simulink model "object_frame_impedance"  (R2025a)
settings: Solver=FixedStepDiscrete  StartTime=0.0  StopTime=inf  FixedStep=0.0315/(4*12)  RelTol=1e-3  EnableMultiTasking=on
undefined symbols (not defined in the file or in its folder): f_step, force_step, K_Conn, K_D, K_Or, K_Ot, K_P, ksi, Kx, l_des, Mo, Newton, qd_initial_touch, R_O_Desired, Raphson, sigbuilder_block, t_f_start, torque_step, x_O_desired
libraries: dspmtrx3 x33, dspinverses x1
(part 6 of 6)

== matlab function object_frame_impedance/Control/IPC/J/J_Or1/Embedded MATLAB Function2 ==
  data: xi input double size=[4 3]; J_r3 output
%#eml
function J_r3 = partial_r3_to_x(xi)


x1 = xi(1,:)';
x2 = xi(2,:)';
x3 = xi(3,:)';
x4 = xi(4,:)';

r1=(( x1-x3 )/norm( x1-x3 ) + ...
    ( x2-x4 )/norm( x2-x4 ));


r1_unit=(r1/norm(r1));

r3 = skew( x1-x3 ) * ( x2-x4 );
r3_unit=r3/norm(r3);

r2_unit = skew(r3_unit)*r1_unit;

% RO=[r1_unit r2_unit r3_unit];


% partial_r3__term1 = (((norm(r3)^2)*eye(3)-(r3)*(r3)') / (norm((r3))^3));
partial_r3__term1 = (-skew(r3)^2)/(norm(r3)^3);

partial_r3__term2_x1x3 = skew(x2-x4)';
partial_r3__term2_x2x4 =  skew(x1-x3); 

partial_r3__term3_x1x2 =  eye(3);
partial_r3__term3_x3x4 = -eye(3);

J_r3_x1 = partial_r3__term1*partial_r3__term2_x1x3*partial_r3__term3_x1x2;

J_r3_x2 = partial_r3__term1*partial_r3__term2_x2x4*partial_r3__term3_x1x2;
       
J_r3_x3 = partial_r3__term1*partial_r3__term2_x1x3*partial_r3__term3_x3x4;
                    
J_r3_x4 = partial_r3__term1*partial_r3__term2_x2x4*partial_r3__term3_x3x4;


J_r3 = [J_r3_x1,J_r3_x2,J_r3_x3,J_r3_x4];

== matlab function object_frame_impedance/Control/IPC/J/J_Or1/Embedded MATLAB Function3 ==
  data: xi input double size=[4 3]; J_r1 output
%#eml
function J_r1 = partial_r1_to_x(xi)


x1 = xi(1,:)';
x2 = xi(2,:)';
x3 = xi(3,:)';
x4 = xi(4,:)';

r1=(( x1-x3 )/norm( x1-x3 ) + ( x2-x4 )/norm( x2-x4 ));

% r1=(( x1-x3 )/norm( x1-x3 ) + ( x2-x4 ))


r1_unit=(r1/norm(r1));

r3= skew( x1-x3 ) * ( x2-x4 );
r3_unit=r3/norm(r3);

r2_unit = skew(r3_unit)*r1_unit;

% RO=[r1_unit r2_unit r3_unit];


% partial_r1__term1 = (((norm(r1)^2)*eye(3)-(r1)*(r1)') / (norm((r1))^3));
partial_r1__term1 = (-skew(r1)^2)/(norm(r1)^3);

partial_r1__term2_x1x3 = (((norm((x1-x3))^2)*eye(3)-(x1-x3)*(x1-x3)') / (norm((x1-x3))^3));
partial_r1__term2_x2x4 = (((norm((x2-x4))^2)*eye(3)-(x2-x4)*(x2-x4)') / (norm((x2-x4))^3));


partial_r1__term3_x1x2 = eye(3);
partial_r1__term3_x3x4 = -eye(3);



J_r1_x1 = partial_r1__term1*partial_r1__term2_x1x3*partial_r1__term3_x1x2;

J_r2 = skew(r3_unit)*J_r1_x1';

J_r1_x2 = partial_r1__term1*partial_r1__term2_x2x4*partial_r1__term3_x1x2;
       
J_r1_x3 = partial_r1__term1*partial_r1__term2_x1x3*partial_r1__term3_x3x4;
       
J_r1_x4 = partial_r1__term1*partial_r1__term2_x2x4*partial_r1__term3_x3x4;


% J_r1_x1 = [partial_r1__term1.*partial_r1__term2_x1x3.*partial_r1__term3_x1x2(:,1), ...
%            partial_r1__term1.*partial_r1__term2_x1x3.*partial_r1__term3_x1x2(:,2), ...
%            partial_r1__term1.*partial_r1__term2_x1x3.*partial_r1__term3_x1x2(:,3)];
% 
% J_r1_x2 = [partial_r1__term1.*partial_r1__term2_x2x4.*partial_r1__term3_x1x2(:,1), ...
%            partial_r1__term1.*partial_r1__term2_x2x4.*partial_r1__term3_x1x2(:,2), ...
%            partial_r1__term1.*partial_r1__term2_x2x4.*partial_r1__term3_x1x2(:,3)];
%        
% J_r1_x3 = [partial_r1__term1.*partial_r1__term2_x1x3.*partial_r1__term3_x3x4(:,1), ...
%            partial_r1__term1.*partial_r1__term2_x1x3.*partial_r1__term3_x3x4(:,2), ...
%            partial_r1__term1.*partial_r1__term2_x1x3.*partial_r1__term3_x3x4(:,3)];
%        
% J_r1_x4 = [partial_r1__term1.*partial_r1__term2_x2x4.*partial_r1__term3_x3x4(:,1), ...
%            partial_r1__term1.*partial_r1__term2_x2x4.*partial_r1__term3_x3x4(:,2), ...
%            partial_r1__term1.*partial_r1__term2_x2x4.*partial_r1__term3_x3x4(:,3)];

J_r1 = [J_r1_x1,J_r1_x2,J_r1_x3,J_r1_x4];

== matlab function object_frame_impedance/Control/IPC/Object Level Damping(theta)/Embedded MATLAB Function ==
  data: q input; M output
%#eml
function M=Inertia_Dynamic_Terms(q)

M1=zeros(16);

L1 = 0.10;
L2 = 1.10;
L3 = 0.60;
L4 = 0.55;

capsule1Inertia = 0.1675;
capsule2Inertia = 0.0837;
capsule3Inertia = 0.0834;

caspule1mass = 2.00;
caspule2mass = 1.00;
caspule3mass = 1.00;

for i=1:4:16,
q1 = q(i);
q2 = q(i+1);
q3 = q(i+2);
q4 = q(i+3);
    
    
M1(i:i+3,i:i+3)=[capsule1Inertia .* cos(q2) .^ 2 + capsule2Inertia .* cos(q2 + q3) ...
   .^ 2 + capsule3Inertia .* cos(q2 + q3 + q4) .^ 2 + caspule1mass  ...
  .* ((1 / 4) .* L2 .^ 2 .* cos(q1) .^ 2 .* cos(q2) .^ 2 + (1 / 4)  ...
  .* L2 .^ 2 .* cos(q2) .^ 2 .* sin(q1) .^ 2) + caspule2mass .* ((( ...
  -1 / 2) .* L3 .* cos(q1) .* cos(q2 + q3) + cos(q1) .* (L2 .* cos( ...
  q2) + L3 .* cos(q2 + q3))) .^ 2 + ((1 / 2) .* L3 .* cos(q2 + q3)  ...
  .* sin(q1) + (-1) .* (L2 .* cos(q2) + L3 .* cos(q2 + q3)) .* sin( ...
  q1)) .^ 2) + caspule3mass .* (((-1 / 2) .* L4 .* cos(q1) .* cos( ...
  q2 + q3 + q4) + cos(q1) .* (L2 .* cos(q2) + L3 .* cos(q2 + q3) +  ...
  L4 .* cos(q2 + q3 + q4))) .^ 2 + ((1 / 2) .* L4 .* cos(q2 + q3 +  ...
  q4) .* sin(q1) + (-1) .* (L2 .* cos(q2) + L3 .* cos(q2 + q3) + L4  ...
  .* cos(q2 + q3 + q4)) .* sin(q1)) .^ 2) + capsule1Inertia .* sin( ...
  q2) .^ 2 + capsule2Inertia .* sin(q2 + q3) .^ 2 + capsule3Inertia  ...
  .* sin(q2 + q3 + q4) .^ 2,caspule2mass .* ((-1) .* ((-1 / 2) .*  ...
  L3 .* cos(q1) .* cos(q2 + q3) + cos(q1) .* (L2 .* cos(q2) + L3 .*  ...
  cos(q2 + q3))) .* sin(q1) .* (L2 .* sin(q2) + (1 / 2) .* L3 .*  ...
  sin(q2 + q3)) + (-1) .* cos(q1) .* ((1 / 2) .* L3 .* cos(q2 + q3)  ...
  .* sin(q1) + (-1) .* (L2 .* cos(q2) + L3 .* cos(q2 + q3)) .* sin( ...
  q1)) .* (L2 .* sin(q2) + (1 / 2) .* L3 .* sin(q2 + q3))) +  ...
  caspule3mass .* ((-1) .* ((-1 / 2) .* L4 .* cos(q1) .* cos(q2 +  ...
  q3 + q4) + cos(q1) .* (L2 .* cos(q2) + L3 .* cos(q2 + q3) + L4 .*  ...
  cos(q2 + q3 + q4))) .* sin(q1) .* (L2 .* sin(q2) + L3 .* sin(q2 +  ...
  q3) + (1 / 2) .* L4 .* sin(q2 + q3 + q4)) + (-1) .* cos(q1) .* (( ...
  1 / 2) .* L4 .* cos(q2 + q3 + q4) .* sin(q1) + (-1) .* (L2 .* cos( ...
  q2) + L3 .* cos(q2 + q3) + L4 .* cos(q2 + q3 + q4)) .* sin(q1)) .* ...
   (L2 .* sin(q2) + L3 .* sin(q2 + q3) + (1 / 2) .* L4 .* sin(q2 +  ...
  q3 + q4))),caspule2mass .* ((-1 / 2) .* L3 .* ((-1 / 2) .* L3 .*  ...
  cos(q1) .* cos(q2 + q3) + cos(q1) .* (L2 .* cos(q2) + L3 .* cos( ...
  q2 + q3))) .* sin(q1) .* sin(q2 + q3) + (-1 / 2) .* L3 .* cos(q1)  ...
  .* ((1 / 2) .* L3 .* cos(q2 + q3) .* sin(q1) + (-1) .* (L2 .* cos( ...
  q2) + L3 .* cos(q2 + q3)) .* sin(q1)) .* sin(q2 + q3)) +  ...
  caspule3mass .* ((-1) .* ((-1 / 2) .* L4 .* cos(q1) .* cos(q2 +  ...
  q3 + q4) + cos(q1) .* (L2 .* cos(q2) + L3 .* cos(q2 + q3) + L4 .*  ...
  cos(q2 + q3 + q4))) .* sin(q1) .* (L3 .* sin(q2 + q3) + (1 / 2) .* ...
   L4 .* sin(q2 + q3 + q4)) + (-1) .* cos(q1) .* ((1 / 2) .* L4 .*  ...
  cos(q2 + q3 + q4) .* sin(q1) + (-1) .* (L2 .* cos(q2) + L3 .* cos( ...
  q2 + q3) + L4 .* cos(q2 + q3 + q4)) .* sin(q1)) .* (L3 .* sin(q2 + ...
   q3) + (1 / 2) .* L4 .* sin(q2 + q3 + q4))),caspule3mass .* ((-1  ...
  / 2) .* L4 .* ((-1 / 2) .* L4 .* cos(q1) .* cos(q2 + q3 + q4) +  ...
  cos(q1) .* (L2 .* cos(q2) + L3 .* cos(q2 + q3) + L4 .* cos(q2 +  ...
  q3 + q4))) .* sin(q1) .* sin(q2 + q3 + q4) + (-1 / 2) .* L4 .*  ...
  cos(q1) .* ((1 / 2) .* L4 .* cos(q2 + q3 + q4) .* sin(q1) + (-1)  ...
  .* (L2 .* cos(q2) + L3 .* cos(q2 + q3) + L4 .* cos(q2 + q3 + q4))  ...
  .* sin(q1)) .* sin(q2 + q3 + q4));caspule2mass .* ((-1) .* ((-1 /  ...
  2) .* L3 .* cos(q1) .* cos(q2 + q3) + cos(q1) .* (L2 .* cos(q2) +  ...
  L3 .* cos(q2 + q3))) .* sin(q1) .* (L2 .* sin(q2) + (1 / 2) .* L3  ...
  .* sin(q2 + q3)) + (-1) .* cos(q1) .* ((1 / 2) .* L3 .* cos(q2 +  ...
  q3) .* sin(q1) + (-1) .* (L2 .* cos(q2) + L3 .* cos(q2 + q3)) .*  ...
  sin(q1)) .* (L2 .* sin(q2) + (1 / 2) .* L3 .* sin(q2 + q3))) +  ...
  caspule3mass .* ((-1) .* ((-1 / 2) .* L4 .* cos(q1) .* cos(q2 +  ...
  q3 + q4) + cos(q1) .* (L2 .* cos(q2) + L3 .* cos(q2 + q3) + L4 .*  ...
  cos(q2 + q3 + q4))) .* sin(q1) .* (L2 .* sin(q2) + L3 .* sin(q2 +  ...
  q3) + (1 / 2) .* L4 .* sin(q2 + q3 + q4)) + (-1) .* cos(q1) .* (( ...
  1 / 2) .* L4 .* cos(q2 + q3 + q4) .* sin(q1) + (-1) .* (L2 .* cos( ...
  q2) + L3 .* cos(q2 + q3) + L4 .* cos(q2 + q3 + q4)) .* sin(q1)) .* ...
   (L2 .* sin(q2) + L3 .* sin(q2 + q3) + (1 / 2) .* L4 .* sin(q2 +  ...
  q3 + q4))),capsule1Inertia .* cos(q1) .^ 2 .* (cos(q1) .^ 2 + sin( ...
  q1) .^ 2) + capsule2Inertia .* cos(q1) .^ 2 .* (cos(q1) .^ 2 +  ...
  sin(q1) .^ 2) + capsule3Inertia .* cos(q1) .^ 2 .* (cos(q1) .^ 2 + ...
   sin(q1) .^ 2) + capsule1Inertia .* sin(q1) .^ 2 .* (cos(q1) .^ 2  ...
  + sin(q1) .^ 2) + capsule2Inertia .* sin(q1) .^ 2 .* (cos(q1) .^  ...
  2 + sin(q1) .^ 2) + capsule3Inertia .* sin(q1) .^ 2 .* (cos(q1)  ...
  .^ 2 + sin(q1) .^ 2) + caspule1mass .* (((1 / 2) .* L2 .* cos(q1)  ...
  .^ 2 .* cos(q2) + (1 / 2) .* L2 .* cos(q2) .* sin(q1) .^ 2) .^ 2 + ...
   (1 / 4) .* L2 .^ 2 .* cos(q1) .^ 2 .* sin(q2) .^ 2 + (1 / 4) .*  ...
  L2 .^ 2 .* sin(q1) .^ 2 .* sin(q2) .^ 2) + caspule2mass .* ((cos( ...
  q1) .* ((-1 / 2) .* L3 .* cos(q1) .* cos(q2 + q3) + cos(q1) .* ( ...
  L2 .* cos(q2) + L3 .* cos(q2 + q3))) + sin(q1) .* ((-1 / 2) .* L3  ...
  .* cos(q2 + q3) .* sin(q1) + (L2 .* cos(q2) + L3 .* cos(q2 + q3))  ...
  .* sin(q1))) .^ 2 + cos(q1) .^ 2 .* (L2 .* sin(q2) + (1 / 2) .*  ...
  L3 .* sin(q2 + q3)) .^ 2 + sin(q1) .^ 2 .* (L2 .* sin(q2) + (1 /  ...
  2) .* L3 .* sin(q2 + q3)) .^ 2) + caspule3mass .* ((cos(q1) .* (( ...
  -1 / 2) .* L4 .* cos(q1) .* cos(q2 + q3 + q4) + cos(q1) .* (L2 .*  ...
  cos(q2) + L3 .* cos(q2 + q3) + L4 .* cos(q2 + q3 + q4))) + sin(q1) ...
   .* ((-1 / 2) .* L4 .* cos(q2 + q3 + q4) .* sin(q1) + (L2 .* cos( ...
  q2) + L3 .* cos(q2 + q3) + L4 .* cos(q2 + q3 + q4)) .* sin(q1)))  ...
  .^ 2 + cos(q1) .^ 2 .* (L2 .* sin(q2) + L3 .* sin(q2 + q3) + (1 /  ...
  2) .* L4 .* sin(q2 + q3 + q4)) .^ 2 + sin(q1) .^ 2 .* (L2 .* sin( ...
  q2) + L3 .* sin(q2 + q3) + (1 / 2) .* L4 .* sin(q2 + q3 + q4)) .^  ...
  2),capsule2Inertia .* cos(q1) .^ 2 .* (cos(q1) .^ 2 + sin(q1) .^  ...
  2) + capsule3Inertia .* cos(q1) .^ 2 .* (cos(q1) .^ 2 + sin(q1)  ...
  .^ 2) + capsule2Inertia .* sin(q1) .^ 2 .* (cos(q1) .^ 2 + sin(q1) ...
   .^ 2) + capsule3Inertia .* sin(q1) .^ 2 .* (cos(q1) .^ 2 + sin( ...
  q1) .^ 2) + caspule2mass .* ((cos(q1) .* ((-1 / 2) .* L3 .* cos( ...
  q1) .* cos(q2 + q3) + cos(q1) .* (L2 .* cos(q2) + L3 .* cos(q2 +  ...
  q3))) + sin(q1) .* ((-1 / 2) .* L3 .* cos(q2 + q3) .* sin(q1) + ( ...
  L2 .* cos(q2) + L3 .* cos(q2 + q3)) .* sin(q1))) .* (cos(q1) .* (( ...
  -1) .* L2 .* cos(q1) .* cos(q2) + (-1 / 2) .* L3 .* cos(q1) .*  ...
  cos(q2 + q3) + cos(q1) .* (L2 .* cos(q2) + L3 .* cos(q2 + q3))) +  ...
  sin(q1) .* ((-1) .* L2 .* cos(q2) .* sin(q1) + (-1 / 2) .* L3 .*  ...
  cos(q2 + q3) .* sin(q1) + (L2 .* cos(q2) + L3 .* cos(q2 + q3)) .*  ...
  sin(q1))) + (1 / 2) .* L3 .* cos(q1) .^ 2 .* sin(q2 + q3) .* (L2  ...
  .* sin(q2) + (1 / 2) .* L3 .* sin(q2 + q3)) + (1 / 2) .* L3 .*  ...
  sin(q1) .^ 2 .* sin(q2 + q3) .* (L2 .* sin(q2) + (1 / 2) .* L3 .*  ...
  sin(q2 + q3))) + caspule3mass .* ((cos(q1) .* ((-1 / 2) .* L4 .*  ...
  cos(q1) .* cos(q2 + q3 + q4) + cos(q1) .* (L2 .* cos(q2) + L3 .*  ...
  cos(q2 + q3) + L4 .* cos(q2 + q3 + q4))) + sin(q1) .* ((-1 / 2) .* ...
   L4 .* cos(q2 + q3 + q4) .* sin(q1) + (L2 .* cos(q2) + L3 .* cos( ...
  q2 + q3) + L4 .* cos(q2 + q3 + q4)) .* sin(q1))) .* (cos(q1) .* (( ...
  -1) .* L2 .* cos(q1) .* cos(q2) + (-1 / 2) .* L4 .* cos(q1) .*  ...
  cos(q2 + q3 + q4) + cos(q1) .* (L2 .* cos(q2) + L3 .* cos(q2 + q3) ...
   + L4 .* cos(q2 + q3 + q4))) + sin(q1) .* ((-1) .* L2 .* cos(q2)  ...
  .* sin(q1) + (-1 / 2) .* L4 .* cos(q2 + q3 + q4) .* sin(q1) + (L2  ...
  .* cos(q2) + L3 .* cos(q2 + q3) + L4 .* cos(q2 + q3 + q4)) .* sin( ...
  q1))) + cos(q1) .^ 2 .* (L3 .* sin(q2 + q3) + (1 / 2) .* L4 .*  ...
  sin(q2 + q3 + q4)) .* (L2 .* sin(q2) + L3 .* sin(q2 + q3) + (1 /  ...
  2) .* L4 .* sin(q2 + q3 + q4)) + sin(q1) .^ 2 .* (L3 .* sin(q2 +  ...
  q3) + (1 / 2) .* L4 .* sin(q2 + q3 + q4)) .* (L2 .* sin(q2) + L3  ...
  .* sin(q2 + q3) + (1 / 2) .* L4 .* sin(q2 + q3 + q4))), ...
  capsule3Inertia .* cos(q1) .^ 2 .* (cos(q1) .^ 2 + sin(q1) .^ 2) + ...
   capsule3Inertia .* sin(q1) .^ 2 .* (cos(q1) .^ 2 + sin(q1) .^ 2)  ...
  + caspule3mass .* ((cos(q1) .* ((-1 / 2) .* L4 .* cos(q1) .* cos( ...
  q2 + q3 + q4) + cos(q1) .* (L2 .* cos(q2) + L3 .* cos(q2 + q3) +  ...
  L4 .* cos(q2 + q3 + q4))) + sin(q1) .* ((-1 / 2) .* L4 .* cos(q2 + ...
   q3 + q4) .* sin(q1) + (L2 .* cos(q2) + L3 .* cos(q2 + q3) + L4 .* ...
   cos(q2 + q3 + q4)) .* sin(q1))) .* (cos(q1) .* ((-1) .* cos(q1)  ...
  .* (L2 .* cos(q2) + L3 .* cos(q2 + q3)) + (-1 / 2) .* L4 .* cos( ...
  q1) .* cos(q2 + q3 + q4) + cos(q1) .* (L2 .* cos(q2) + L3 .* cos( ...
  q2 + q3) + L4 .* cos(q2 + q3 + q4))) + sin(q1) .* ((-1) .* (L2 .*  ...
  cos(q2) + L3 .* cos(q2 + q3)) .* sin(q1) + (-1 / 2) .* L4 .* cos( ...
  q2 + q3 + q4) .* sin(q1) + (L2 .* cos(q2) + L3 .* cos(q2 + q3) +  ...
  L4 .* cos(q2 + q3 + q4)) .* sin(q1))) + (1 / 2) .* L4 .* cos(q1)  ...
  .^ 2 .* sin(q2 + q3 + q4) .* (L2 .* sin(q2) + L3 .* sin(q2 + q3) + ...
   (1 / 2) .* L4 .* sin(q2 + q3 + q4)) + (1 / 2) .* L4 .* sin(q1)  ...
  .^ 2 .* sin(q2 + q3 + q4) .* (L2 .* sin(q2) + L3 .* sin(q2 + q3) + ...
   (1 / 2) .* L4 .* sin(q2 + q3 + q4)));caspule2mass .* ((-1 / 2) .* ...
   L3 .* ((-1 / 2) .* L3 .* cos(q1) .* cos(q2 + q3) + cos(q1) .* ( ...
  L2 .* cos(q2) + L3 .* cos(q2 + q3))) .* sin(q1) .* sin(q2 + q3) +  ...
  (-1 / 2) .* L3 .* cos(q1) .* ((1 / 2) .* L3 .* cos(q2 + q3) .*  ...
  sin(q1) + (-1) .* (L2 .* cos(q2) + L3 .* cos(q2 + q3)) .* sin(q1)) ...
   .* sin(q2 + q3)) + caspule3mass .* ((-1) .* ((-1 / 2) .* L4 .*  ...
  cos(q1) .* cos(q2 + q3 + q4) + cos(q1) .* (L2 .* cos(q2) + L3 .*  ...
  cos(q2 + q3) + L4 .* cos(q2 + q3 + q4))) .* sin(q1) .* (L3 .* sin( ...
  q2 + q3) + (1 / 2) .* L4 .* sin(q2 + q3 + q4)) + (-1) .* cos(q1)  ...
  .* ((1 / 2) .* L4 .* cos(q2 + q3 + q4) .* sin(q1) + (-1) .* (L2 .* ...
   cos(q2) + L3 .* cos(q2 + q3) + L4 .* cos(q2 + q3 + q4)) .* sin( ...
  q1)) .* (L3 .* sin(q2 + q3) + (1 / 2) .* L4 .* sin(q2 + q3 + q4))) ...
  ,capsule2Inertia .* cos(q1) .^ 2 .* (cos(q1) .^ 2 + sin(q1) .^ 2)  ...
  + capsule3Inertia .* cos(q1) .^ 2 .* (cos(q1) .^ 2 + sin(q1) .^ 2) ...
   + capsule2Inertia .* sin(q1) .^ 2 .* (cos(q1) .^ 2 + sin(q1) .^  ...
  2) + capsule3Inertia .* sin(q1) .^ 2 .* (cos(q1) .^ 2 + sin(q1)  ...
  .^ 2) + caspule2mass .* ((cos(q1) .* ((-1 / 2) .* L3 .* cos(q1) .* ...
   cos(q2 + q3) + cos(q1) .* (L2 .* cos(q2) + L3 .* cos(q2 + q3))) + ...
   sin(q1) .* ((-1 / 2) .* L3 .* cos(q2 + q3) .* sin(q1) + (L2 .*  ...
  cos(q2) + L3 .* cos(q2 + q3)) .* sin(q1))) .* (cos(q1) .* ((-1) .* ...
   L2 .* cos(q1) .* cos(q2) + (-1 / 2) .* L3 .* cos(q1) .* cos(q2 +  ...
  q3) + cos(q1) .* (L2 .* cos(q2) + L3 .* cos(q2 + q3))) + sin(q1)  ...
  .* ((-1) .* L2 .* cos(q2) .* sin(q1) + (-1 / 2) .* L3 .* cos(q2 +  ...
  q3) .* sin(q1) + (L2 .* cos(q2) + L3 .* cos(q2 + q3)) .* sin(q1))) ...
   + (1 / 2) .* L3 .* cos(q1) .^ 2 .* sin(q2 + q3) .* (L2 .* sin(q2) ...
   + (1 / 2) .* L3 .* sin(q2 + q3)) + (1 / 2) .* L3 .* sin(q1) .^ 2  ...
  .* sin(q2 + q3) .* (L2 .* sin(q2) + (1 / 2) .* L3 .* sin(q2 + q3)) ...
  ) + caspule3mass .* ((cos(q1) .* ((-1 / 2) .* L4 .* cos(q1) .*  ...
  cos(q2 + q3 + q4) + cos(q1) .* (L2 .* cos(q2) + L3 .* cos(q2 + q3) ...
   + L4 .* cos(q2 + q3 + q4))) + sin(q1) .* ((-1 / 2) .* L4 .* cos( ...
  q2 + q3 + q4) .* sin(q1) + (L2 .* cos(q2) + L3 .* cos(q2 + q3) +  ...
  L4 .* cos(q2 + q3 + q4)) .* sin(q1))) .* (cos(q1) .* ((-1) .* L2  ...
  .* cos(q1) .* cos(q2) + (-1 / 2) .* L4 .* cos(q1) .* cos(q2 + q3 + ...
   q4) + cos(q1) .* (L2 .* cos(q2) + L3 .* cos(q2 + q3) + L4 .* cos( ...
  q2 + q3 + q4))) + sin(q1) .* ((-1) .* L2 .* cos(q2) .* sin(q1) + ( ...
  -1 / 2) .* L4 .* cos(q2 + q3 + q4) .* sin(q1) + (L2 .* cos(q2) +  ...
  L3 .* cos(q2 + q3) + L4 .* cos(q2 + q3 + q4)) .* sin(q1))) + cos( ...
  q1) .^ 2 .* (L3 .* sin(q2 + q3) + (1 / 2) .* L4 .* sin(q2 + q3 +  ...
  q4)) .* (L2 .* sin(q2) + L3 .* sin(q2 + q3) + (1 / 2) .* L4 .*  ...
  sin(q2 + q3 + q4)) + sin(q1) .^ 2 .* (L3 .* sin(q2 + q3) + (1 / 2) ...
   .* L4 .* sin(q2 + q3 + q4)) .* (L2 .* sin(q2) + L3 .* sin(q2 +  ...
  q3) + (1 / 2) .* L4 .* sin(q2 + q3 + q4))),capsule2Inertia .* cos( ...
  q1) .^ 2 .* (cos(q1) .^ 2 + sin(q1) .^ 2) + capsule3Inertia .*  ...
  cos(q1) .^ 2 .* (cos(q1) .^ 2 + sin(q1) .^ 2) + capsule2Inertia .* ...
   sin(q1) .^ 2 .* (cos(q1) .^ 2 + sin(q1) .^ 2) + capsule3Inertia  ...
  .* sin(q1) .^ 2 .* (cos(q1) .^ 2 + sin(q1) .^ 2) + caspule2mass .* ...
   ((cos(q1) .* ((-1) .* L2 .* cos(q1) .* cos(q2) + (-1 / 2) .* L3  ...
  .* cos(q1) .* cos(q2 + q3) + cos(q1) .* (L2 .* cos(q2) + L3 .*  ...
  cos(q2 + q3))) + sin(q1) .* ((-1) .* L2 .* cos(q2) .* sin(q1) + ( ...
  -1 / 2) .* L3 .* cos(q2 + q3) .* sin(q1) + (L2 .* cos(q2) + L3 .*  ...
  cos(q2 + q3)) .* sin(q1))) .^ 2 + (1 / 4) .* L3 .^ 2 .* cos(q1)  ...
  .^ 2 .* sin(q2 + q3) .^ 2 + (1 / 4) .* L3 .^ 2 .* sin(q1) .^ 2 .*  ...
  sin(q2 + q3) .^ 2) + caspule3mass .* ((cos(q1) .* ((-1) .* L2 .*  ...
  cos(q1) .* cos(q2) + (-1 / 2) .* L4 .* cos(q1) .* cos(q2 + q3 +  ...
  q4) + cos(q1) .* (L2 .* cos(q2) + L3 .* cos(q2 + q3) + L4 .* cos( ...
  q2 + q3 + q4))) + sin(q1) .* ((-1) .* L2 .* cos(q2) .* sin(q1) + ( ...
  -1 / 2) .* L4 .* cos(q2 + q3 + q4) .* sin(q1) + (L2 .* cos(q2) +  ...
  L3 .* cos(q2 + q3) + L4 .* cos(q2 + q3 + q4)) .* sin(q1))) .^ 2 +  ...
  cos(q1) .^ 2 .* (L3 .* sin(q2 + q3) + (1 / 2) .* L4 .* sin(q2 +  ...
  q3 + q4)) .^ 2 + sin(q1) .^ 2 .* (L3 .* sin(q2 + q3) + (1 / 2) .*  ...
  L4 .* sin(q2 + q3 + q4)) .^ 2),capsule3Inertia .* cos(q1) .^ 2 .*  ...
  (cos(q1) .^ 2 + sin(q1) .^ 2) + capsule3Inertia .* sin(q1) .^ 2 .* ...
   (cos(q1) .^ 2 + sin(q1) .^ 2) + caspule3mass .* ((cos(q1) .* (( ...
  -1) .* L2 .* cos(q1) .* cos(q2) + (-1 / 2) .* L4 .* cos(q1) .*  ...
  cos(q2 + q3 + q4) + cos(q1) .* (L2 .* cos(q2) + L3 .* cos(q2 + q3) ...
   + L4 .* cos(q2 + q3 + q4))) + sin(q1) .* ((-1) .* L2 .* cos(q2)  ...
  .* sin(q1) + (-1 / 2) .* L4 .* cos(q2 + q3 + q4) .* sin(q1) + (L2  ...
  .* cos(q2) + L3 .* cos(q2 + q3) + L4 .* cos(q2 + q3 + q4)) .* sin( ...
  q1))) .* (cos(q1) .* ((-1) .* cos(q1) .* (L2 .* cos(q2) + L3 .*  ...
  cos(q2 + q3)) + (-1 / 2) .* L4 .* cos(q1) .* cos(q2 + q3 + q4) +  ...
  cos(q1) .* (L2 .* cos(q2) + L3 .* cos(q2 + q3) + L4 .* cos(q2 +  ...
  q3 + q4))) + sin(q1) .* ((-1) .* (L2 .* cos(q2) + L3 .* cos(q2 +  ...
  q3)) .* sin(q1) + (-1 / 2) .* L4 .* cos(q2 + q3 + q4) .* sin(q1) + ...
   (L2 .* cos(q2) + L3 .* cos(q2 + q3) + L4 .* cos(q2 + q3 + q4)) .* ...
   sin(q1))) + (1 / 2) .* L4 .* cos(q1) .^ 2 .* sin(q2 + q3 + q4) .* ...
   (L3 .* sin(q2 + q3) + (1 / 2) .* L4 .* sin(q2 + q3 + q4)) + (1 /  ...
  2) .* L4 .* sin(q1) .^ 2 .* sin(q2 + q3 + q4) .* (L3 .* sin(q2 +  ...
  q3) + (1 / 2) .* L4 .* sin(q2 + q3 + q4)));caspule3mass .* ((-1 /  ...
  2) .* L4 .* ((-1 / 2) .* L4 .* cos(q1) .* cos(q2 + q3 + q4) + cos( ...
  q1) .* (L2 .* cos(q2) + L3 .* cos(q2 + q3) + L4 .* cos(q2 + q3 +  ...
  q4))) .* sin(q1) .* sin(q2 + q3 + q4) + (-1 / 2) .* L4 .* cos(q1)  ...
  .* ((1 / 2) .* L4 .* cos(q2 + q3 + q4) .* sin(q1) + (-1) .* (L2 .* ...
   cos(q2) + L3 .* cos(q2 + q3) + L4 .* cos(q2 + q3 + q4)) .* sin( ...
  q1)) .* sin(q2 + q3 + q4)),capsule3Inertia .* cos(q1) .^ 2 .* ( ...
  cos(q1) .^ 2 + sin(q1) .^ 2) + capsule3Inertia .* sin(q1) .^ 2 .*  ...
  (cos(q1) .^ 2 + sin(q1) .^ 2) + caspule3mass .* ((cos(q1) .* ((-1  ...
  / 2) .* L4 .* cos(q1) .* cos(q2 + q3 + q4) + cos(q1) .* (L2 .*  ...
  cos(q2) + L3 .* cos(q2 + q3) + L4 .* cos(q2 + q3 + q4))) + sin(q1) ...
   .* ((-1 / 2) .* L4 .* cos(q2 + q3 + q4) .* sin(q1) + (L2 .* cos( ...
  q2) + L3 .* cos(q2 + q3) + L4 .* cos(q2 + q3 + q4)) .* sin(q1)))  ...
  .* (cos(q1) .* ((-1) .* cos(q1) .* (L2 .* cos(q2) + L3 .* cos(q2 + ...
   q3)) + (-1 / 2) .* L4 .* cos(q1) .* cos(q2 + q3 + q4) + cos(q1)  ...
  .* (L2 .* cos(q2) + L3 .* cos(q2 + q3) + L4 .* cos(q2 + q3 + q4))) ...
   + sin(q1) .* ((-1) .* (L2 .* cos(q2) + L3 .* cos(q2 + q3)) .*  ...
  sin(q1) + (-1 / 2) .* L4 .* cos(q2 + q3 + q4) .* sin(q1) + (L2 .*  ...
  cos(q2) + L3 .* cos(q2 + q3) + L4 .* cos(q2 + q3 + q4)) .* sin(q1) ...
  )) + (1 / 2) .* L4 .* cos(q1) .^ 2 .* sin(q2 + q3 + q4) .* (L2 .*  ...
  sin(q2) + L3 .* sin(q2 + q3) + (1 / 2) .* L4 .* sin(q2 + q3 + q4)) ...
   + (1 / 2) .* L4 .* sin(q1) .^ 2 .* sin(q2 + q3 + q4) .* (L2 .*  ...
  sin(q2) + L3 .* sin(q2 + q3) + (1 / 2) .* L4 .* sin(q2 + q3 + q4)) ...
  ),capsule3Inertia .* cos(q1) .^ 2 .* (cos(q1) .^ 2 + sin(q1) .^ 2) ...
   + capsule3Inertia .* sin(q1) .^ 2 .* (cos(q1) .^ 2 + sin(q1) .^  ...
  2) + caspule3mass .* ((cos(q1) .* ((-1) .* L2 .* cos(q1) .* cos( ...
  q2) + (-1 / 2) .* L4 .* cos(q1) .* cos(q2 + q3 + q4) + cos(q1) .*  ...
  (L2 .* cos(q2) + L3 .* cos(q2 + q3) + L4 .* cos(q2 + q3 + q4))) +  ...
  sin(q1) .* ((-1) .* L2 .* cos(q2) .* sin(q1) + (-1 / 2) .* L4 .*  ...
  cos(q2 + q3 + q4) .* sin(q1) + (L2 .* cos(q2) + L3 .* cos(q2 + q3) ...
   + L4 .* cos(q2 + q3 + q4)) .* sin(q1))) .* (cos(q1) .* ((-1) .*  ...
  cos(q1) .* (L2 .* cos(q2) + L3 .* cos(q2 + q3)) + (-1 / 2) .* L4  ...
  .* cos(q1) .* cos(q2 + q3 + q4) + cos(q1) .* (L2 .* cos(q2) + L3  ...
  .* cos(q2 + q3) + L4 .* cos(q2 + q3 + q4))) + sin(q1) .* ((-1) .*  ...
  (L2 .* cos(q2) + L3 .* cos(q2 + q3)) .* sin(q1) + (-1 / 2) .* L4  ...
  .* cos(q2 + q3 + q4) .* sin(q1) + (L2 .* cos(q2) + L3 .* cos(q2 +  ...
  q3) + L4 .* cos(q2 + q3 + q4)) .* sin(q1))) + (1 / 2) .* L4 .*  ...
  cos(q1) .^ 2 .* sin(q2 + q3 + q4) .* (L3 .* sin(q2 + q3) + (1 / 2) ...
   .* L4 .* sin(q2 + q3 + q4)) + (1 / 2) .* L4 .* sin(q1) .^ 2 .*  ...
  sin(q2 + q3 + q4) .* (L3 .* sin(q2 + q3) + (1 / 2) .* L4 .* sin( ...
  q2 + q3 + q4))),capsule3Inertia .* cos(q1) .^ 2 .* (cos(q1) .^ 2 + ...
   sin(q1) .^ 2) + capsule3Inertia .* sin(q1) .^ 2 .* (cos(q1) .^ 2  ...
  + sin(q1) .^ 2) + caspule3mass .* ((cos(q1) .* ((-1) .* cos(q1) .* ...
   (L2 .* cos(q2) + L3 .* cos(q2 + q3)) + (-1 / 2) .* L4 .* cos(q1)  ...
  .* cos(q2 + q3 + q4) + cos(q1) .* (L2 .* cos(q2) + L3 .* cos(q2 +  ...
  q3) + L4 .* cos(q2 + q3 + q4))) + sin(q1) .* ((-1) .* (L2 .* cos( ...
  q2) + L3 .* cos(q2 + q3)) .* sin(q1) + (-1 / 2) .* L4 .* cos(q2 +  ...
  q3 + q4) .* sin(q1) + (L2 .* cos(q2) + L3 .* cos(q2 + q3) + L4 .*  ...
  cos(q2 + q3 + q4)) .* sin(q1))) .^ 2 + (1 / 4) .* L4 .^ 2 .* cos( ...
  q1) .^ 2 .* sin(q2 + q3 + q4) .^ 2 + (1 / 4) .* L4 .^ 2 .* sin(q1) ...
   .^ 2 .* sin(q2 + q3 + q4) .^ 2)];
end
M=M1;

== matlab function object_frame_impedance/Control/IPC/J/Embedded MATLAB Function1 ==
  data: xi input double size=[4 3]; RO output
%#eml
function RO=R_O(xi)



x1 = xi(1,:);
x2 = xi(2,:);
x3 = xi(3,:);
x4 = xi(4,:);

% r1=( xi(1,:)-xi(3,:) )/norm( xi(1,:)-xi(3,:) ) + ...
%     ( xi(2,:)-xi(4,:) )/norm( xi(2,:)-xi(4,:) );

r1=( x1-x3 )/norm( x1-x3 ) + ...
    ( x2-x4 )/norm( x2-x4 );


r1_unit=r1/norm(r1);

% r3= cross( (x1-x3),( x2-x4 ))';

r3= skew( x1-x3 ) * ( x2-x4 )';
r3_unit=r3/norm(r3);

r2_unit = skew(r3_unit)*r1_unit';

l=[r1_unit' r2_unit r3_unit];
RO=l;

== matlab function object_frame_impedance/Control/IPC/Object Level Damping(theta)/Embedded MATLAB Function1 ==
  data: u input; y output
function y = fcn(u)
%#eml

y = inv(u);

== matlab function object_frame_impedance/Control/IPC/J/J_Ot1/Embedded MATLAB Function ==
  data: u input; y output
function y = fcn(u)
%#eml

y = (u(1,:)+u(2,:)+u(3,:)+u(4,:))/4;

== matlab function object_frame_impedance/Control/IPC/J/J_Ot1/Embedded MATLAB Function1 ==
  data: v_in input size=[3 1]; S output
%#eml
function S = skew(v_in)

v=v_in';
    S = [  0   -v(1,3)  v(1,2);
          v(1,3)  0    -v(1,1);
          -v(1,2) v(1,1)   0];

== matlab function object_frame_impedance/Control/IPC/J/J_Or1/Embedded MATLAB Function ==
  data: u input size=[3 3]; y output
function y = fcn(u)
%#eml

y = u(:,1)';

== matlab function object_frame_impedance/Control/IPC/J/J_Or1/Embedded MATLAB Function4 ==
  data: u input size=[3 3]; y output
function y = fcn(u)
%#eml

y = u(:,2)';
